simulink model "ControleFF"  (R2020a)
settings: Solver=FixedStepAuto  StartTime=0.0  StopTime=9  FixedStep=1/100  RelTol=1e-3
values from neighbouring files (symbols this model uses):
  Beff = 50    [controle.m]    (also in controle_FF.m; controle_PD.m)
  Jeff = 2.2    [controle.m]    (also in controle_FF.m = 0.5; controle_PD.m = 0.5)
  K = 17.7    [controle.m]    (also in controle_FF.m = 0.785398163397; controle_PD.m = 0.785398163397)
  Kd = (2*zeta*wn*Jeff - Beff)/K    (= -2.32768361582)    [controle.m]    (also in controle_FF.m = -44.5633840657; controle_PD.m = -44.5633840657)
  Kp = (wn^2*Jeff)/K    (= 0.497175141243)    [controle.m]    (also in controle_FF.m = 143.239448783; controle_PD.m = 143.239448783)
  N = 10    [controle.m]    (also in controle_FF.m = 3; controle_PD.m = 3)
  r = 1/100    (= 0.01)    [controle.m]    (also in controle_FF.m = 1./[231.22*4 139.138 139.138 231.22 231.22]; controle_PD.m = 1./[231.22*4 139.138 139.138 231.22 231.22])
  SP_theta = [0;0;0;0;0]    [controle.m]    (also in controle_FF.m = [0 0 0 0 0]; controle_PD.m)
  thdotdotpath = [0 0 0 0 0]    [controle_FF.m]
  thdotpath = [0 0 0 0 0]    [controle_FF.m]
  thpath = [0 0 0 0 0]    [controle_FF.m]
libraries: simulink_extras x6
(part 1 of 2)
settings Model: Creator=Karoline  LastModifiedBy=lunet
settings DataIOCC: ReturnWorkspaceOutputs=off
settings DebuggingCC: ArithmeticOperatorsInVariantConditions=warning
settings SFSimCC: SimUseLocalCustomCode=off  CustomCodeUndefinedFunction=UseInterfaceOnly
settings RTWCC: RTWUseLocalCustomCode=off
settings CodeAppCC: StateflowObjectComments=on

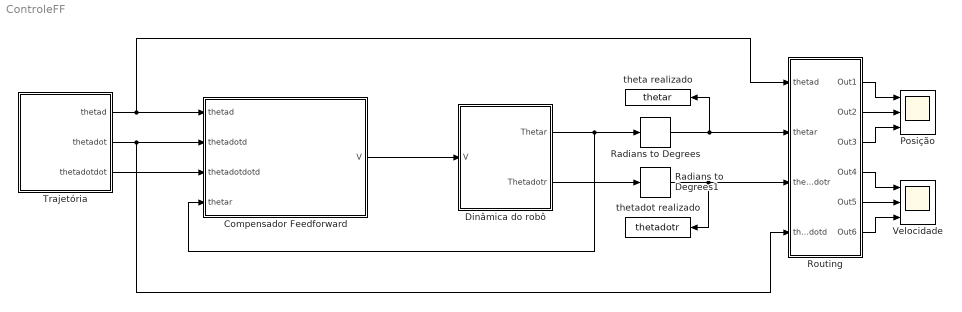
== system ControleFF ==
  Compensador Feedforward : Subsystem
  Dinâmica do robô : Subsystem
  Posição : Scope  NumInputPorts=3
  Radians to Degrees : simulink_extras/Transformations/Radians to Degrees
  Radians to Degrees1 : simulink_extras/Transformations/Radians to Degrees
  Routing : Subsystem
  Trajetória : Subsystem
  Velocidade : Scope  NumInputPorts=3
  theta realizado : ToWorkspace  VariableName=thetar  SaveFormat=Structure With Time  SampleTime=-1
  thetadot realizado : ToWorkspace  VariableName=thetadotr  SaveFormat=Structure With Time  SampleTime=-1
  wires:
  Radians to Degrees/1 -> theta realizado/1, Routing/2(thetar)
  Dinâmica do robô/2("Thetadotr ") -> Radians to Degrees1/1
  Dinâmica do robô/1(Thetar) -> Radians to Degrees/1, Compensador Feedforward/4(thetar)
  Radians to Degrees1/1 -> thetadot realizado/1, Routing/3(thetadotr)
  Compensador Feedforward/1(V) -> Dinâmica do robô/1(V)
  Trajetória/1(thetad) -> Routing/1(thetad), Compensador Feedforward/1(thetad)
  Trajetória/2(thetadot) -> Routing/4(thetadotd), Compensador Feedforward/2(thetadotd)
  Trajetória/3(thetadotdot) -> Compensador Feedforward/3(thetadotdotd)
  Routing/1(Out1) -> Posição/1
  Routing/2(Out2) -> Posição/2
  Routing/3(Out3) -> Posição/3
  Routing/4(Out4) -> Velocidade/1
  Routing/5(Out5) -> Velocidade/2
  Routing/6(Out6) -> Velocidade/3

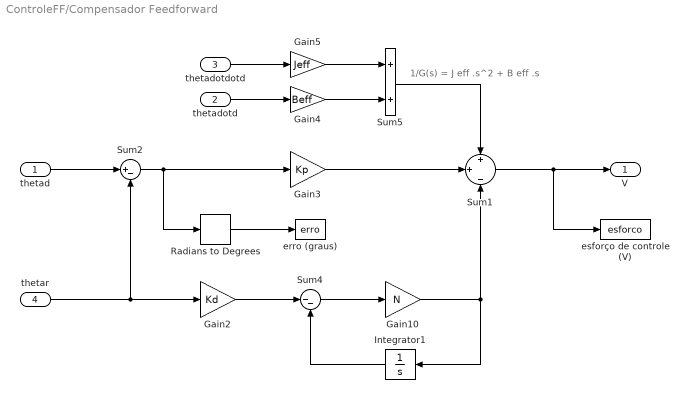
== system ControleFF/Compensador Feedforward ==
  note: 1/G(s) = J eff .s^2 + B eff .s
  thetad : Inport
  thetadotd : Inport  Port=2
  thetadotdotd : Inport  Port=3
  thetar : Inport  Port=4
  Gain10 : Gain  Gain=N
  Gain2 : Gain  Gain=Kd
  Gain3 : Gain  Gain=Kp
  Gain4 : Gain  Gain=Beff
  Gain5 : Gain  Gain=Jeff
  Integrator1 : Integrator
  Radians to Degrees : simulink_extras/Transformations/Radians to Degrees
  Sum1 : Sum  Inputs=+|+|-
  Sum2 : Sum  Inputs=|+-
  Sum4 : Sum  Inputs=|--
  Sum5 : Sum
  erro (graus) : ToWorkspace  VariableName=erro  SaveFormat=Structure With Time  SampleTime=-1
  esforço de controle (V) : ToWorkspace  VariableName=esforco  SaveFormat=Structure With Time  SampleTime=-1
  V : Outport  VectorParamsAs1DForOutWhenUnconnected=off
  wires:
  Gain2/1 -> Sum4/1
  thetar/1 -> Sum2/2, Gain2/1
  Sum4/1 -> Gain10/1
  Sum2/1 -> Radians to Degrees/1, Gain3/1
  Radians to Degrees/1 -> erro (graus)/1
  thetad/1 -> Sum2/1
  Integrator1/1 -> Sum4/2
  Gain10/1 -> Sum1/3, Integrator1/1
  Gain3/1 -> Sum1/2
  Sum1/1 -> esforço de controle (V)/1, V/1
  Gain4/1 -> Sum5/2
  Sum5/1 -> Sum1/1
  thetadotd/1 -> Gain4/1
  thetadotdotd/1 -> Gain5/1
  Gain5/1 -> Sum5/1

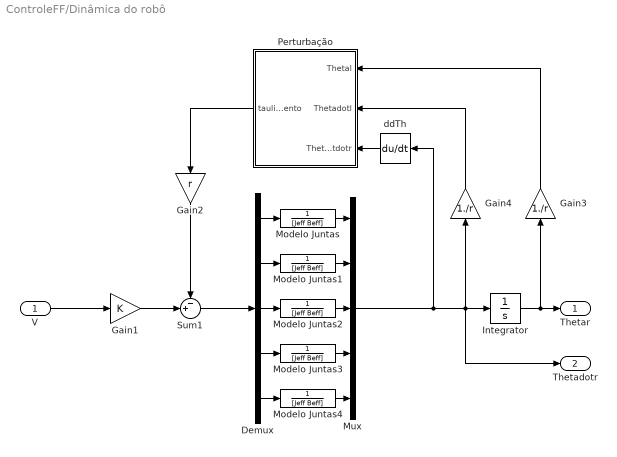
== system ControleFF/Dinâmica do robô ==
  V : Inport
  Demux : Demux  Outputs=5
  Gain1 : Gain  Gain=K
  Gain2 : Gain  Gain=r
  Gain3 : Gain  Gain=1./r
  Gain4 : Gain  Gain=1./r
  Integrator : Integrator  InitialCondition=SP_theta*pi/180
  Modelo Juntas{,1..4} (5 alike) : TransferFcn  Denominator=[Jeff Beff]
  Mux : Mux  Inputs=5
  Perturbação : Subsystem
  Sum1 : Sum  Inputs=-+|
  ddTh : Derivative
  Thetar : Outport  VectorParamsAs1DForOutWhenUnconnected=off
  "Thetadotr " : Outport  Port=2  VectorParamsAs1DForOutWhenUnconnected=off
  wires:
  Perturbação/1(tauligamento) -> Gain2/1
  Gain1/1 -> Sum1/2
  Sum1/1 -> Demux/1
  Integrator/1 -> Thetar/1, Gain3/1
  V/1 -> Gain1/1
  Gain2/1 -> Sum1/1
  Mux/1 -> ddTh/1, Gain4/1, Integrator/1, "Thetadotr "/1
  ddTh/1 -> Perturbação/3(Thetadotdotr)
  Gain3/1 -> Perturbação/1(Thetal)
  Gain4/1 -> Perturbação/2(Thetadotl)
  Demux/4 -> Modelo Juntas3/1
  Demux/2 -> Modelo Juntas1/1
  Modelo Juntas/1 -> Mux/1
  Demux/3 -> Modelo Juntas2/1
  Demux/5 -> Modelo Juntas4/1
  Modelo Juntas4/1 -> Mux/5
  Modelo Juntas2/1 -> Mux/3
  Demux/1 -> Modelo Juntas/1
  Modelo Juntas3/1 -> Mux/4
  Modelo Juntas1/1 -> Mux/2

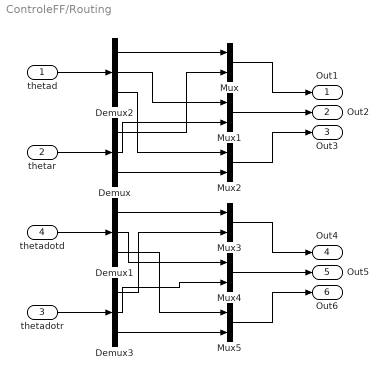
== system ControleFF/Routing ==
  thetad : Inport
  thetar : Inport  Port=2
  thetadotr : Inport  Port=3
  thetadotd : Inport  Port=4
  Demux{,1..3} (4 alike) : Demux  Outputs=3
  Mux{,1..5} (6 alike) : Mux  Inputs=2
  Out1 : Outport  VectorParamsAs1DForOutWhenUnconnected=off
  Out2 : Outport  Port=2  VectorParamsAs1DForOutWhenUnconnected=off
  Out3 : Outport  Port=3  VectorParamsAs1DForOutWhenUnconnected=off
  Out4 : Outport  Port=4  VectorParamsAs1DForOutWhenUnconnected=off
  Out5 : Outport  Port=5  VectorParamsAs1DForOutWhenUnconnected=off
  Out6 : Outport  Port=6  VectorParamsAs1DForOutWhenUnconnected=off
  wires:
  Demux2/2 -> Mux1/1
  Demux/2 -> Mux1/2
  Demux2/1 -> Mux/1
  Demux1/3 -> Mux5/1
  Demux3/2 -> Mux4/2
  Demux1/1 -> Mux3/1
  Demux/1 -> Mux/2
  Demux3/1 -> Mux3/2
  Mux1/1 -> Out2/1
  Demux2/3 -> Mux2/1
  Mux4/1 -> Out5/1
  Demux3/3 -> Mux5/2
  Demux1/2 -> Mux4/1
  Demux/3 -> Mux2/2
  Mux3/1 -> Out4/1
  Mux/1 -> Out1/1
  Mux5/1 -> Out6/1
  thetadotr/1 -> Demux3/1
  thetad/1 -> Demux2/1
  thetadotd/1 -> Demux1/1
  Mux2/1 -> Out3/1
  thetar/1 -> Demux/1

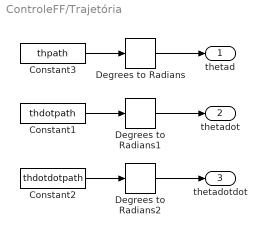
== system ControleFF/Trajetória ==
  Constant1 : Constant  Value=thdotpath  VectorParams1D=off
  Constant2 : Constant  Value=thdotdotpath  VectorParams1D=off
  Constant3 : Constant  Value=thpath  VectorParams1D=off
  Degrees to Radians : simulink_extras/Transformations/Degrees to Radians
  Degrees to Radians1 : simulink_extras/Transformations/Degrees to Radians
  Degrees to Radians2 : simulink_extras/Transformations/Degrees to Radians
  thetad : Outport  VectorParamsAs1DForOutWhenUnconnected=off
  thetadot : Outport  Port=2  VectorParamsAs1DForOutWhenUnconnected=off
  thetadotdot : Outport  Port=3  VectorParamsAs1DForOutWhenUnconnected=off
  wires:
  Degrees to Radians/1 -> thetad/1
  Constant3/1 -> Degrees to Radians/1
  Degrees to Radians1/1 -> thetadot/1
  Degrees to Radians2/1 -> thetadotdot/1
  Constant2/1 -> Degrees to Radians2/1
  Constant1/1 -> Degrees to Radians1/1

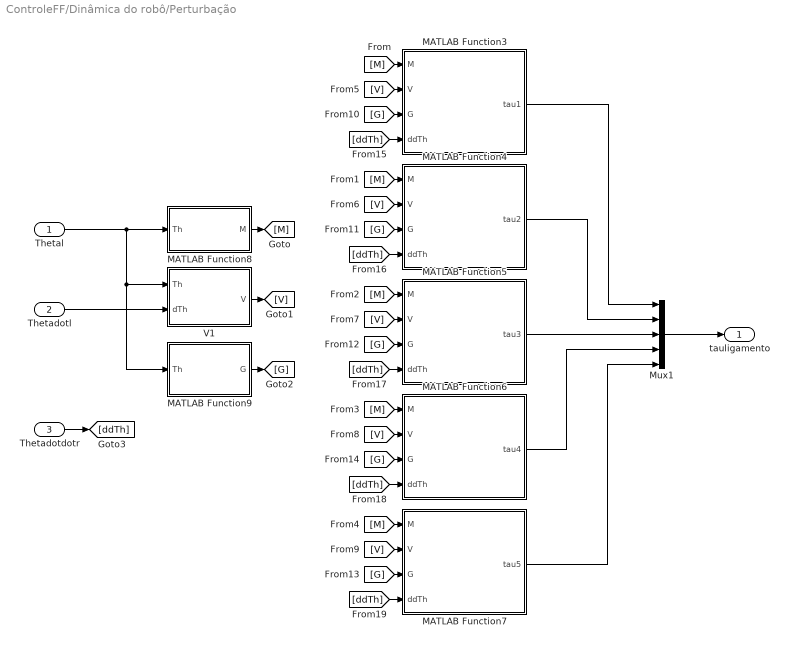
== system ControleFF/Dinâmica do robô/Perturbação ==
  Thetal : Inport
  Thetadotl : Inport  Port=2
  Thetadotdotr : Inport  Port=3
  MATLAB Function3 : MATLAB Function  TreatAsAtomicUnit=on
  MATLAB Function4 : MATLAB Function  TreatAsAtomicUnit=on
  MATLAB Function5 : MATLAB Function  TreatAsAtomicUnit=on
  MATLAB Function6 : MATLAB Function  TreatAsAtomicUnit=on
  MATLAB Function7 : MATLAB Function  TreatAsAtomicUnit=on
  MATLAB Function8 : MATLAB Function  TreatAsAtomicUnit=on
  MATLAB Function9 : MATLAB Function  TreatAsAtomicUnit=on
  Mux1 : Mux  Inputs=5
  V1 : MATLAB Function  TreatAsAtomicUnit=on
  tauligamento : Outport  VectorParamsAs1DForOutWhenUnconnected=off
  wires:
  [G] -> MATLAB Function6/3(G)
  MATLAB Function8/1(M) -> [M]
  [M] -> MATLAB Function6/1(M)
  [M] -> MATLAB Function4/1(M)
  [M] -> MATLAB Function3/1(M)
  Thetal/1 -> MATLAB Function8/1(Th), MATLAB Function9/1(Th), V1/1(Th)
  [ddTh] -> MATLAB Function5/4(ddTh)
  [V] -> MATLAB Function3/2(V)
  [ddTh] -> MATLAB Function3/4(ddTh)
  [G] -> MATLAB Function7/3(G)
  [ddTh] -> MATLAB Function6/4(ddTh)
  [V] -> MATLAB Function6/2(V)
  Thetadotl/1 -> V1/2(dTh)
  [G] -> MATLAB Function5/3(G)
  [G] -> MATLAB Function3/3(G)
  [G] -> MATLAB Function4/3(G)
  MATLAB Function9/1(G) -> [G]
  [V] -> MATLAB Function7/2(V)
  [ddTh] -> MATLAB Function4/4(ddTh)
  [V] -> MATLAB Function5/2(V)
  [V] -> MATLAB Function4/2(V)
  V1/1(V) -> [V]
  [M] -> MATLAB Function7/1(M)
  [M] -> MATLAB Function5/1(M)
  [ddTh] -> MATLAB Function7/4(ddTh)
  Mux1/1 -> tauligamento/1
  MATLAB Function3/1(tau1) -> Mux1/1
  MATLAB Function4/1(tau2) -> Mux1/2
  MATLAB Function5/1(tau3) -> Mux1/3
  MATLAB Function6/1(tau4) -> Mux1/4
  MATLAB Function7/1(tau5) -> Mux1/5
  Thetadotdotr/1 -> [ddTh]

== matlab function ControleFF/Dinâmica do robô/Perturbação/MATLAB Function3 ==
  data: M input; V input; tau1 output; G input; ddTh input
function tau1  = calcul_dk1(M, V, G, ddTh)

tau1 = M(1,2)*ddTh(2) + M(1,3)*ddTh(3) + M(1,4)*ddTh(4) + M(1,5)*ddTh(5) ...
       + V(1) + G(1);

== matlab function ControleFF/Dinâmica do robô/Perturbação/MATLAB Function4 ==
  data: M input; V input; tau2 output; G input; ddTh input
function tau2  = calcul_dk2(M, V, G, ddTh)

tau2 = M(2,1)*ddTh(1) + M(2,3)*ddTh(3) + M(2,4)*ddTh(4) + M(2,5)*ddTh(5) ...
       + V(2) + G(2);

== matlab function ControleFF/Dinâmica do robô/Perturbação/MATLAB Function5 ==
  data: M input; V input; tau3 output; G input; ddTh input
function tau3  = calcul_dk3(M, V, G, ddTh)

tau3 = M(3,1)*ddTh(1) + M(3,2)*ddTh(2) + M(3,4)*ddTh(4) + M(3,5)*ddTh(5) ...
       + V(3) + G(3);

== matlab function ControleFF/Dinâmica do robô/Perturbação/MATLAB Function6 ==
  data: M input; V input; tau4 output; G input; ddTh input
function tau4 = calcul_dk4(M, V, G, ddTh)

tau4 = M(4,1)*ddTh(1) + M(4,2)*ddTh(2) + M(4,3)*ddTh(3) + M(4,5)*ddTh(5) ...
       + V(4) + G(4);

== matlab function ControleFF/Dinâmica do robô/Perturbação/MATLAB Function7 ==
  data: M input; V input; tau5 output; G input; ddTh input
function tau5  = calcul_dk5(M, V, G, ddTh)

tau5 = M(5,1)*ddTh(1) + M(5,2)*ddTh(2) + M(5,3)*ddTh(3) + M(5,4)*ddTh(4) ...
       + V(5) + G(5);

== matlab function ControleFF/Dinâmica do robô/Perturbação/MATLAB Function8 ==
  data: Th input; M output
function M = calcul_M(Th)

th1 = Th(1);
th2 = Th(2);
th3 = Th(3);
th4 = Th(4);
th5 = Th(5);

M = [ (87*cos(th2)^2*cos(th5))/2500 + (87*cos(th3)^2*cos(th5))/2500 - (33*cos(th2)^2*sin(th3))/50 + (53231*cos(th2)^2)/62500 + (8453*cos(th3)^2)/31250 - (9*cos(th5)^2)/3200 - (8453*cos(th2)^2*cos(th3)^2)/15625 - (217*cos(th2)^2*cos(th4)^2)/80000 + (9*cos(th2)^2*cos(th5)^2)/3200 - (217*cos(th3)^2*cos(th4)^2)/80000 + (9*cos(th3)^2*cos(th5)^2)/3200 - (87*cos(th2)^2*cos(th3)^2*cos(th5))/1250 - (33*cos(th2)*cos(th3)*sin(th2))/50 + (217*cos(th2)^2*cos(th3)^2*cos(th4)^2)/40000 - (9*cos(th2)^2*cos(th3)^2*cos(th5)^2)/1600 + (9*cos(th2)^2*cos(th4)^2*cos(th5)^2)/3200 + (9*cos(th3)^2*cos(th4)^2*cos(th5)^2)/3200 - (3*cos(th2)^2*cos(th5)*sin(th3))/80 - (9*cos(th2)^2*cos(th3)^2*cos(th4)^2*cos(th5)^2)/1600 - (3*cos(th2)*cos(th3)*cos(th5)*sin(th2))/80 + (8453*cos(th2)*cos(th3)*sin(th2)*sin(th3))/15625 - (87*cos(th2)*cos(th4)*sin(th2)*sin(th5))/2500 - (87*cos(th3)*cos(th4)*sin(th3)*sin(th5))/2500 - (3*cos(th2)^2*cos(th3)*cos(th4)*sin(th5))/80 + (3*cos(th2)*cos(th4)*sin(th2)*sin(th3)*sin(th5))/80 - (217*cos(th2)*cos(th3)*cos(th4)^2*sin(th2)*sin(th3))/40000 + (9*cos(th2)*cos(th3)*cos(th5)^2*sin(th2)*sin(th3))/1600 + (87*cos(th2)*cos(th3)^2*cos(th4)*sin(th2)*sin(th5))/1250 + (87*cos(th2)^2*cos(th3)*cos(th4)*sin(th3)*sin(th5))/1250 + (87*cos(th2)*cos(th3)*cos(th5)*sin(th2)*sin(th3))/1250 - (9*cos(th2)*cos(th4)*cos(th5)*sin(th2)*sin(th5))/1600 - (9*cos(th3)*cos(th4)*cos(th5)*sin(th3)*sin(th5))/1600 + (9*cos(th2)*cos(th3)*cos(th4)^2*cos(th5)^2*sin(th2)*sin(th3))/1600 + (9*cos(th2)*cos(th3)^2*cos(th4)*cos(th5)*sin(th2)*sin(th5))/800 + (9*cos(th2)^2*cos(th3)*cos(th4)*cos(th5)*sin(th3)*sin(th5))/800 + 3793/80000, -(sin(th4)*(1500*sin(th2)*sin(th5) - 217*cos(th2)*cos(th4)*sin(th3) - 217*cos(th3)*cos(th4)*sin(th2) + 1392*cos(th2)*cos(th3)*sin(th5) - 1392*sin(th2)*sin(th3)*sin(th5) + 225*cos(th2)*cos(th3)*cos(th5)*sin(th5) - 225*cos(th5)*sin(th2)*sin(th3)*sin(th5) + 225*cos(th2)*cos(th4)*cos(th5)^2*sin(th3) + 225*cos(th3)*cos(th4)*cos(th5)^2*sin(th2)))/80000, (sin(th4)*(217*cos(th2)*cos(th4)*sin(th3) + 217*cos(th3)*cos(th4)*sin(th2) - 1392*cos(th2)*cos(th3)*sin(th5) + 1392*sin(th2)*sin(th3)*sin(th5) - 225*cos(th2)*cos(th3)*cos(th5)*sin(th5) + 225*cos(th5)*sin(th2)*sin(th3)*sin(th5) - 225*cos(th2)*cos(th4)*cos(th5)^2*sin(th3) - 225*cos(th3)*cos(th4)*cos(th5)^2*sin(th2)))/80000, (489*cos(th2)*cos(th3))/80000 - (489*sin(th2)*sin(th3))/80000 - (3*cos(th2)*cos(th4)*sin(th5))/160 - (9*cos(th2)*cos(th3)*cos(th5)^2)/3200 + (9*cos(th5)^2*sin(th2)*sin(th3))/3200 + (87*cos(th2)*cos(th4)*sin(th3)*sin(th5))/5000 + (87*cos(th3)*cos(th4)*sin(th2)*sin(th5))/5000 + (9*cos(th2)*cos(th4)*cos(th5)*sin(th3)*sin(th5))/3200 + (9*cos(th3)*cos(th4)*cos(th5)*sin(th2)*sin(th5))/3200, (sin(th4)*(353*cos(th2)*sin(th3) + 353*cos(th3)*sin(th2) - 1500*cos(th2)*cos(th5) + 1392*cos(th2)*cos(th5)*sin(th3) + 1392*cos(th3)*cos(th5)*sin(th2)))/80000;
                                                                                                                                                                                                                                                                                                                                                                                                                                                                                                                                                                                                                                                                                                                                                                                                                                                                                                                                                                                                                                                                                                                                                                                                                                                                                                                                                                                                                                                                                                                                                                                            -(sin(th4)*(1500*sin(th2)*sin(th5) - 217*cos(th2)*cos(th4)*sin(th3) - 217*cos(th3)*cos(th4)*sin(th2) + 1392*cos(th2)*cos(th3)*sin(th5) - 1392*sin(th2)*sin(th3)*sin(th5) + 225*cos(th2)*cos(th3)*cos(th5)*sin(th5) - 225*cos(th5)*sin(th2)*sin(th3)*sin(th5) + 225*cos(th2)*cos(th4)*cos(th5)^2*sin(th3) + 225*cos(th3)*cos(th4)*cos(th5)^2*sin(th2)))/80000,                                                                                                                                                                                                                       (87*cos(th5))/2500 - (33*sin(th3))/50 - (3*cos(th5)*sin(th3))/80 + (217*cos(th4)^2)/80000 + (9*cos(th5)^2)/3200 - (9*cos(th4)^2*cos(th5)^2)/3200 - (3*cos(th3)*cos(th4)*sin(th5))/80 + 54781/62500,                                                                                                                                                                                   (87*cos(th5))/2500 - (33*sin(th3))/100 - (3*cos(th5)*sin(th3))/160 + (217*cos(th4)^2)/80000 + (9*cos(th5)^2)/3200 - (9*cos(th4)^2*cos(th5)^2)/3200 - (3*cos(th3)*cos(th4)*sin(th5))/160 + 72749/250000,                                                                                                                                                                                                                                                                                                                                                                                                                     -(3*sin(th4)*sin(th5)*(75*cos(th5) - 500*sin(th3) + 464))/80000,                                                          (353*cos(th4))/80000 - (3*cos(th3)*sin(th5))/160 + (87*cos(th4)*cos(th5))/5000 - (3*cos(th4)*cos(th5)*sin(th3))/160;
                                                                                                                                                                                                                                                                                                                                                                                                                                                                                                                                                                                                                                                                                                                                                                                                                                                                                                                                                                                                                                                                                                                                                                                                                                                                                                                                                                                                                                                                                                                                                                                                                            (sin(th4)*(217*cos(th2)*cos(th4)*sin(th3) + 217*cos(th3)*cos(th4)*sin(th2) - 1392*cos(th2)*cos(th3)*sin(th5) + 1392*sin(th2)*sin(th3)*sin(th5) - 225*cos(th2)*cos(th3)*cos(th5)*sin(th5) + 225*cos(th5)*sin(th2)*sin(th3)*sin(th5) - 225*cos(th2)*cos(th4)*cos(th5)^2*sin(th3) - 225*cos(th3)*cos(th4)*cos(th5)^2*sin(th2)))/80000,                                                                                                                                                                                                                   (87*cos(th5))/2500 - (33*sin(th3))/100 - (3*cos(th5)*sin(th3))/160 + (217*cos(th4)^2)/80000 + (9*cos(th5)^2)/3200 - (9*cos(th4)^2*cos(th5)^2)/3200 - (3*cos(th3)*cos(th4)*sin(th5))/160 + 72749/250000,                                                                                                                                                                                                                                                                                          (87*cos(th5))/2500 + (217*cos(th4)^2)/80000 + (9*cos(th5)^2)/3200 - (9*cos(th4)^2*cos(th5)^2)/3200 + 72749/250000,                                                                                                                                                                                                                                                                                                                                                                                                                                       -(3*sin(th4)*sin(th5)*(75*cos(th5) + 464))/80000,                                                                                                                                                         (cos(th4)*(1392*cos(th5) + 353))/80000;
                                                                                                                                                                                                                                                                                                                                                                                                                                                                                                                                                                                                                                                                                                                                                                                                                                                                                                                                                                                                                                                                                                                                                                                                                                                                                                                                                                                                                                                                                                                                                      (489*cos(th2)*cos(th3))/80000 - (489*sin(th2)*sin(th3))/80000 - (3*cos(th2)*cos(th4)*sin(th5))/160 - (9*cos(th2)*cos(th3)*cos(th5)^2)/3200 + (9*cos(th5)^2*sin(th2)*sin(th3))/3200 + (87*cos(th2)*cos(th4)*sin(th3)*sin(th5))/5000 + (87*cos(th3)*cos(th4)*sin(th2)*sin(th5))/5000 + (9*cos(th2)*cos(th4)*cos(th5)*sin(th3)*sin(th5))/3200 + (9*cos(th3)*cos(th4)*cos(th5)*sin(th2)*sin(th5))/3200,                                                                                                                                                                                                                                                                                                                                                                               -(3*sin(th4)*sin(th5)*(75*cos(th5) - 500*sin(th3) + 464))/80000,                                                                                                                                                                                                                                                                                                                                                                 -(3*sin(th4)*sin(th5)*(75*cos(th5) + 464))/80000,                                                                                                                                                                                                                                                                                                                                                                                                                                                              489/80000 - (9*cos(th5)^2)/3200,                                                                                                                                                                                                    0;
                                                                                                                                                                                                                                                                                                                                                                                                                                                                                                                                                                                                                                                                                                                                                                                                                                                                                                                                                                                                                                                                                                                                                                                                                                                                                                                                                                                                                                                                                                                                                                                                                                                                                                                                                                                                                                                 (sin(th4)*(353*cos(th2)*sin(th3) + 353*cos(th3)*sin(th2) - 1500*cos(th2)*cos(th5) + 1392*cos(th2)*cos(th5)*sin(th3) + 1392*cos(th3)*cos(th5)*sin(th2)))/80000,                                                                                                                                                                                                                                                                                                               (353*cos(th4))/80000 - (3*cos(th3)*sin(th5))/160 + (87*cos(th4)*cos(th5))/5000 - (3*cos(th4)*cos(th5)*sin(th3))/160,                                                                                                                                                                                                                                                                                                                                                                              (cos(th4)*(1392*cos(th5) + 353))/80000,                                                                                                                                                                                                                                                                                                                                                                                                                                                                                               0,                                                                                                                                                                                            353/80000];

== matlab function ControleFF/Dinâmica do robô/Perturbação/MATLAB Function9 ==
  data: Th input; G output
function G = calcul_G(Th)

g = 9.80665;
th1 = Th(1);
th2 = Th(2);
th3 = Th(3);
th4 = Th(4);
th5 = Th(5);

G = [                                                                                                                                                                                                                                                                                               0;
 -g*((49*cos(th2)*sin(th3))/125 - cos(th2)/2 + (49*cos(th3)*sin(th2))/125 + (3*cos(th2)*cos(th5)*sin(th3))/40 + (3*cos(th3)*cos(th5)*sin(th2))/40 + (3*cos(th2)*cos(th3)*cos(th4)*sin(th5))/40 - (3*cos(th4)*sin(th2)*sin(th3)*sin(th5))/40);
                 -g*((49*cos(th2)*sin(th3))/125 + (49*cos(th3)*sin(th2))/125 + (3*cos(th2)*cos(th5)*sin(th3))/40 + (3*cos(th3)*cos(th5)*sin(th2))/40 + (3*cos(th2)*cos(th3)*cos(th4)*sin(th5))/40 - (3*cos(th4)*sin(th2)*sin(th3)*sin(th5))/40);
                                                                                                                                                                                                                                                (3*g*sin(th4)*sin(th5)*sin(th2 + th3))/40;
                                                                                       -g*((3*cos(th2)*cos(th3)*sin(th5))/40 - (3*sin(th2)*sin(th3)*sin(th5))/40 + (3*cos(th2)*cos(th4)*cos(th5)*sin(th3))/40 + (3*cos(th3)*cos(th4)*cos(th5)*sin(th2))/40)];
